simulink model "UART"  (R2025a)
settings: Solver=FixedStepAuto  StartTime=0.0  StopTime=10  FixedStep=1e-6  RelTol=1e-3
undefined symbols (not defined in the file): Bit_1, Bit_2, Bit_3, Bit_4, Bit_5, Bit_6, Bit_7, Bit_8
libraries: simulink_extras x158, fl_lib x17, nesl_utility x8, simulink x7
(part 2 of 6)

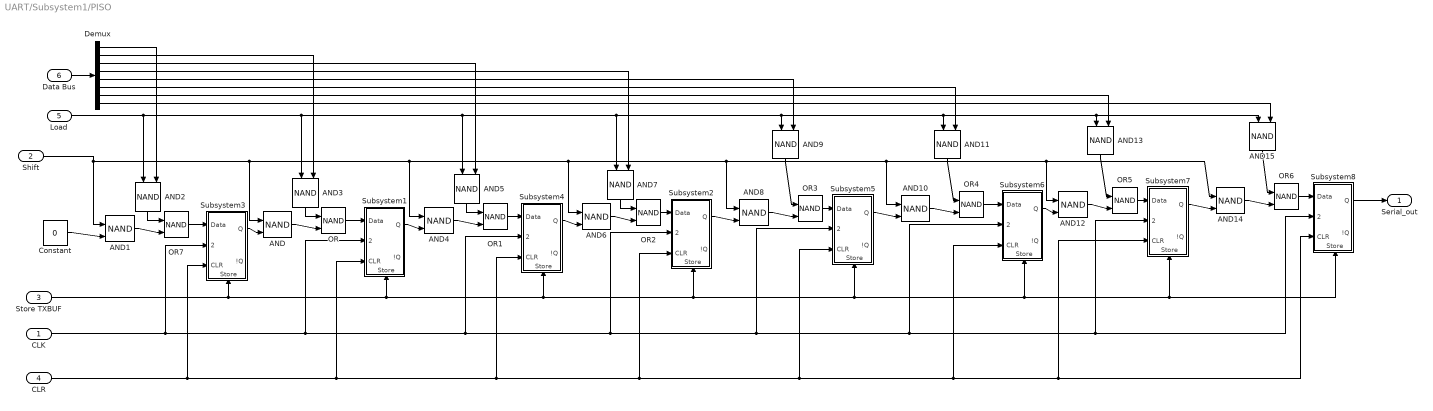
== system UART/Subsystem1/PISO ==
  "CLK " : Inport
  Shift : Inport  Port=2
  Store TXBUF : Inport  Port=3
  "CLR " : Inport  Port=4
  Load : Inport  Port=5
  Data Bus : Inport  Port=6
  AND{,1..15} (16 alike) : Logic  Operator=NAND  IconShape=distinctive  AllPortsSameDT=off  OutDataTypeStr=boolean
  Constant : Constant  Value=0
  Demux : Demux  Outputs=8
  OR{,1..7} (8 alike) : Logic  Operator=NAND  IconShape=distinctive  AllPortsSameDT=off  OutDataTypeStr=boolean
  Subsystem1 : Subsystem
      settings: PortSchema="{\"entries\":[{\"content\":{\"sides\":[{\"content\":{\"connectorIds\":[\"In1\",\"In2\",\"In3\"]},\"type\":\"ConnectorPlacement.EquallySpacedRectSide\",\"uuid\":\"7f3c85a8-435a-48c3-b59c-f5d5714c847e\"},{\"content\":{\"connectorIds\":[\"Out1\",\"Out2\"],\"side\":\"RIGHT\"},\"type\":\"ConnectorPlacement.EquallySpacedRectSide\",\"uuid\":\"17207f13-8340-45d6-91b4-1610668ce323\"},{\"content\":{\"side\":\"TOP\"},\"type\":\"ConnectorPlacement.EquallySpacedRectSide\",\"uuid\":\"04d61695-a4c9-4852-a4b1-2cdbdbfa921f\"},{\"content\":{\"connectorIds\":[\"In4\"],\"side\":\"BOTTOM\"},\"type\":\"ConnectorPlacement.EquallySpacedRectSide\",\"uuid\":\"a1770489-59eb-478b-9b54-00148a18765c\"}]},\"type\":\"ConnectorPlacement.EquallySpacedConnector\",\"uuid\":\"06dc9f9c-9f45-42f3-b967-f8303bc685fc\"}],\"packageUris\":[\"http://schema.mathworks.com/mf0/Connector/R2020b\"],\"version\":\"1.0\"}"
  Subsystem2 : Subsystem
      settings: PortSchema="{\"entries\":[{\"content\":{\"sides\":[{\"content\":{\"connectorIds\":[\"In1\",\"In2\",\"In3\"]},\"type\":\"ConnectorPlacement.EquallySpacedRectSide\",\"uuid\":\"7f3c85a8-435a-48c3-b59c-f5d5714c847e\"},{\"content\":{\"connectorIds\":[\"Out1\",\"Out2\"],\"side\":\"RIGHT\"},\"type\":\"ConnectorPlacement.EquallySpacedRectSide\",\"uuid\":\"17207f13-8340-45d6-91b4-1610668ce323\"},{\"content\":{\"side\":\"TOP\"},\"type\":\"ConnectorPlacement.EquallySpacedRectSide\",\"uuid\":\"04d61695-a4c9-4852-a4b1-2cdbdbfa921f\"},{\"content\":{\"connectorIds\":[\"In4\"],\"side\":\"BOTTOM\"},\"type\":\"ConnectorPlacement.EquallySpacedRectSide\",\"uuid\":\"a1770489-59eb-478b-9b54-00148a18765c\"}]},\"type\":\"ConnectorPlacement.EquallySpacedConnector\",\"uuid\":\"06dc9f9c-9f45-42f3-b967-f8303bc685fc\"}],\"packageUris\":[\"http://schema.mathworks.com/mf0/Connector/R2020b\"],\"version\":\"1.0\"}"
  Subsystem3 : Subsystem
      settings: PortSchema="{\"entries\":[{\"content\":{\"sides\":[{\"content\":{\"connectorIds\":[\"In1\",\"In2\",\"In3\"]},\"type\":\"ConnectorPlacement.EquallySpacedRectSide\",\"uuid\":\"7f3c85a8-435a-48c3-b59c-f5d5714c847e\"},{\"content\":{\"connectorIds\":[\"Out1\",\"Out2\"],\"side\":\"RIGHT\"},\"type\":\"ConnectorPlacement.EquallySpacedRectSide\",\"uuid\":\"17207f13-8340-45d6-91b4-1610668ce323\"},{\"content\":{\"side\":\"TOP\"},\"type\":\"ConnectorPlacement.EquallySpacedRectSide\",\"uuid\":\"04d61695-a4c9-4852-a4b1-2cdbdbfa921f\"},{\"content\":{\"connectorIds\":[\"In4\"],\"side\":\"BOTTOM\"},\"type\":\"ConnectorPlacement.EquallySpacedRectSide\",\"uuid\":\"a1770489-59eb-478b-9b54-00148a18765c\"}]},\"type\":\"ConnectorPlacement.EquallySpacedConnector\",\"uuid\":\"06dc9f9c-9f45-42f3-b967-f8303bc685fc\"}],\"packageUris\":[\"http://schema.mathworks.com/mf0/Connector/R2020b\"],\"version\":\"1.0\"}"
  Subsystem4 : Subsystem
      settings: PortSchema="{\"entries\":[{\"content\":{\"sides\":[{\"content\":{\"connectorIds\":[\"In1\",\"In2\",\"In3\"]},\"type\":\"ConnectorPlacement.EquallySpacedRectSide\",\"uuid\":\"7f3c85a8-435a-48c3-b59c-f5d5714c847e\"},{\"content\":{\"connectorIds\":[\"Out1\",\"Out2\"],\"side\":\"RIGHT\"},\"type\":\"ConnectorPlacement.EquallySpacedRectSide\",\"uuid\":\"17207f13-8340-45d6-91b4-1610668ce323\"},{\"content\":{\"side\":\"TOP\"},\"type\":\"ConnectorPlacement.EquallySpacedRectSide\",\"uuid\":\"04d61695-a4c9-4852-a4b1-2cdbdbfa921f\"},{\"content\":{\"connectorIds\":[\"In4\"],\"side\":\"BOTTOM\"},\"type\":\"ConnectorPlacement.EquallySpacedRectSide\",\"uuid\":\"a1770489-59eb-478b-9b54-00148a18765c\"}]},\"type\":\"ConnectorPlacement.EquallySpacedConnector\",\"uuid\":\"06dc9f9c-9f45-42f3-b967-f8303bc685fc\"}],\"packageUris\":[\"http://schema.mathworks.com/mf0/Connector/R2020b\"],\"version\":\"1.0\"}"
  Subsystem5 : Subsystem
      settings: PortSchema="{\"entries\":[{\"content\":{\"sides\":[{\"content\":{\"connectorIds\":[\"In1\",\"In2\",\"In3\"]},\"type\":\"ConnectorPlacement.EquallySpacedRectSide\",\"uuid\":\"7f3c85a8-435a-48c3-b59c-f5d5714c847e\"},{\"content\":{\"connectorIds\":[\"Out1\",\"Out2\"],\"side\":\"RIGHT\"},\"type\":\"ConnectorPlacement.EquallySpacedRectSide\",\"uuid\":\"17207f13-8340-45d6-91b4-1610668ce323\"},{\"content\":{\"side\":\"TOP\"},\"type\":\"ConnectorPlacement.EquallySpacedRectSide\",\"uuid\":\"04d61695-a4c9-4852-a4b1-2cdbdbfa921f\"},{\"content\":{\"connectorIds\":[\"In4\"],\"side\":\"BOTTOM\"},\"type\":\"ConnectorPlacement.EquallySpacedRectSide\",\"uuid\":\"a1770489-59eb-478b-9b54-00148a18765c\"}]},\"type\":\"ConnectorPlacement.EquallySpacedConnector\",\"uuid\":\"06dc9f9c-9f45-42f3-b967-f8303bc685fc\"}],\"packageUris\":[\"http://schema.mathworks.com/mf0/Connector/R2020b\"],\"version\":\"1.0\"}"
  Subsystem6 : Subsystem
      settings: PortSchema="{\"entries\":[{\"content\":{\"sides\":[{\"content\":{\"connectorIds\":[\"In1\",\"In2\",\"In3\"]},\"type\":\"ConnectorPlacement.EquallySpacedRectSide\",\"uuid\":\"7f3c85a8-435a-48c3-b59c-f5d5714c847e\"},{\"content\":{\"connectorIds\":[\"Out1\",\"Out2\"],\"side\":\"RIGHT\"},\"type\":\"ConnectorPlacement.EquallySpacedRectSide\",\"uuid\":\"17207f13-8340-45d6-91b4-1610668ce323\"},{\"content\":{\"side\":\"TOP\"},\"type\":\"ConnectorPlacement.EquallySpacedRectSide\",\"uuid\":\"04d61695-a4c9-4852-a4b1-2cdbdbfa921f\"},{\"content\":{\"connectorIds\":[\"In4\"],\"side\":\"BOTTOM\"},\"type\":\"ConnectorPlacement.EquallySpacedRectSide\",\"uuid\":\"a1770489-59eb-478b-9b54-00148a18765c\"}]},\"type\":\"ConnectorPlacement.EquallySpacedConnector\",\"uuid\":\"06dc9f9c-9f45-42f3-b967-f8303bc685fc\"}],\"packageUris\":[\"http://schema.mathworks.com/mf0/Connector/R2020b\"],\"version\":\"1.0\"}"
  Subsystem7 : Subsystem
      settings: PortSchema="{\"entries\":[{\"content\":{\"sides\":[{\"content\":{\"connectorIds\":[\"In1\",\"In2\",\"In3\"]},\"type\":\"ConnectorPlacement.EquallySpacedRectSide\",\"uuid\":\"7f3c85a8-435a-48c3-b59c-f5d5714c847e\"},{\"content\":{\"connectorIds\":[\"Out1\",\"Out2\"],\"side\":\"RIGHT\"},\"type\":\"ConnectorPlacement.EquallySpacedRectSide\",\"uuid\":\"17207f13-8340-45d6-91b4-1610668ce323\"},{\"content\":{\"side\":\"TOP\"},\"type\":\"ConnectorPlacement.EquallySpacedRectSide\",\"uuid\":\"04d61695-a4c9-4852-a4b1-2cdbdbfa921f\"},{\"content\":{\"connectorIds\":[\"In4\"],\"side\":\"BOTTOM\"},\"type\":\"ConnectorPlacement.EquallySpacedRectSide\",\"uuid\":\"a1770489-59eb-478b-9b54-00148a18765c\"}]},\"type\":\"ConnectorPlacement.EquallySpacedConnector\",\"uuid\":\"06dc9f9c-9f45-42f3-b967-f8303bc685fc\"}],\"packageUris\":[\"http://schema.mathworks.com/mf0/Connector/R2020b\"],\"version\":\"1.0\"}"
  Subsystem8 : Subsystem
      settings: PortSchema="{\"entries\":[{\"content\":{\"sides\":[{\"content\":{\"connectorIds\":[\"In1\",\"In2\",\"In3\"]},\"type\":\"ConnectorPlacement.EquallySpacedRectSide\",\"uuid\":\"7f3c85a8-435a-48c3-b59c-f5d5714c847e\"},{\"content\":{\"connectorIds\":[\"Out1\",\"Out2\"],\"side\":\"RIGHT\"},\"type\":\"ConnectorPlacement.EquallySpacedRectSide\",\"uuid\":\"17207f13-8340-45d6-91b4-1610668ce323\"},{\"content\":{\"side\":\"TOP\"},\"type\":\"ConnectorPlacement.EquallySpacedRectSide\",\"uuid\":\"04d61695-a4c9-4852-a4b1-2cdbdbfa921f\"},{\"content\":{\"connectorIds\":[\"In4\"],\"side\":\"BOTTOM\"},\"type\":\"ConnectorPlacement.EquallySpacedRectSide\",\"uuid\":\"a1770489-59eb-478b-9b54-00148a18765c\"}]},\"type\":\"ConnectorPlacement.EquallySpacedConnector\",\"uuid\":\"06dc9f9c-9f45-42f3-b967-f8303bc685fc\"}],\"packageUris\":[\"http://schema.mathworks.com/mf0/Connector/R2020b\"],\"version\":\"1.0\"}"
  Serial_out : Outport
  wires:
  AND12/1 -> OR5/2
  AND14/1 -> OR6/2
  AND13/1 -> OR5/1
  OR6/1 -> Subsystem8/1(Data)
  AND6/1 -> OR2/2
  AND7/1 -> OR2/1
  Subsystem4/1(Q) -> AND6/2
  OR2/1 -> Subsystem2/1(Data)
  Subsystem2/1(Q) -> AND8/2
  AND15/1 -> OR6/1
  AND8/1 -> OR3/2
  AND3/1 -> OR/1
  OR5/1 -> Subsystem7/1(Data)
  Subsystem7/1(Q) -> AND14/2
  AND11/1 -> OR4/1
  AND9/1 -> OR3/1
  Subsystem6/1(Q) -> AND12/2
  OR3/1 -> Subsystem5/1(Data)
  OR4/1 -> Subsystem6/1(Data)
  OR1/1 -> Subsystem4/1(Data)
  AND5/1 -> OR1/1
  AND/1 -> OR/2
  AND4/1 -> OR1/2
  Subsystem1/1(Q) -> AND4/2
  Subsystem3/1(Q) -> AND/2
  OR/1 -> Subsystem1/1(Data)
  OR7/1 -> Subsystem3/1(Data)
  Subsystem5/1(Q) -> AND10/2
  AND10/1 -> OR4/2
  Data Bus/1 -> Demux/1
  AND2/1 -> OR7/1
  AND1/1 -> OR7/2
  Shift/1 -> AND1/1, AND6/1, AND10/1, AND12/1, AND14/1, AND8/1, AND4/1, AND/1
  Subsystem8/1(Q) -> Serial_out/1
  Store TXBUF/1 -> Subsystem3/4(Store), Subsystem1/4(Store), Subsystem4/4(Store), Subsystem2/4(Store), Subsystem5/4(Store), Subsystem6/4(Store), Subsystem8/4(Store), Subsystem7/4(Store)
  "CLK "/1 -> Subsystem3/2(Clock), Subsystem1/2(Clock), Subsystem4/2(Clock), Subsystem2/2(Clock), Subsystem5/2(Clock), Subsystem6/2(Clock), Subsystem8/2(Clock), Subsystem7/2(Clock)
  "CLR "/1 -> Subsystem3/3(CLR), Subsystem1/3(CLR), Subsystem4/3(CLR), Subsystem2/3(CLR), Subsystem5/3(CLR), Subsystem6/3(CLR), Subsystem8/3(CLR), Subsystem7/3(CLR)
  Constant/1 -> AND1/2
  Load/1 -> AND2/1, AND3/1, AND5/1, AND7/1, AND9/1, AND11/1, AND13/1, AND15/1
  Demux/1 -> AND2/2
  Demux/2 -> AND3/2
  Demux/3 -> AND5/2
  Demux/4 -> AND7/2
  Demux/5 -> AND9/2
  Demux/6 -> AND11/2
  Demux/7 -> AND13/2
  Demux/8 -> AND15/2

== system UART/Subsystem1/RX Counter ==
  BC_Reset : Inport
  INC : Inport  Port=2
  Constant : Constant
  D Flip-Flop{5..7,11} (4 alike) : simulink_extras/Flip Flops/D Flip-Flop
  Delay One Step : Delay  DelayLength=1
  Demux : Demux
  Half Adder : Subsystem
      settings: PortSchema="{\"entries\":[{\"content\":{\"sides\":[{\"content\":{\"connectorIds\":[\"In1\"]},\"type\":\"ConnectorPlacement.EquallySpacedRectSide\",\"uuid\":\"d3a7e232-15f2-47a9-a065-9480c81dc57e\"},{\"content\":{\"connectorIds\":[\"Out1\"],\"side\":\"RIGHT\"},\"type\":\"ConnectorPlacement.EquallySpacedRectSide\",\"uuid\":\"e118f150-fee7-4aeb-941e-53c3f02c6791\"},{\"content\":{\"connectorIds\":[\"Out2\"],\"side\":\"TOP\"},\"type\":\"ConnectorPlacement.EquallySpacedRectSide\",\"uuid\":\"6d9038ab-faad-455b-a9c5-8fe0bbf34e51\"},{\"content\":{\"connectorIds\":[\"In2\"],\"side\":\"BOTTOM\"},\"type\":\"ConnectorPlacement.EquallySpacedRectSide\",\"uuid\":\"d09c8d4f-08f3-4c52-88a6-8c6db517fc7a\"}]},\"type\":\"ConnectorPlacement.EquallySpacedConnector\",\"uuid\":\"5bc947ce-f1cd-4957-9186-40c14c78de7d\"}],\"packageUris\":[\"http://schema.mathworks.com/mf0/Connector/R2020b\"],\"version\":\"1.0\"}"
  Half Adder1 : Subsystem
      settings: PortSchema="{\"entries\":[{\"content\":{\"sides\":[{\"content\":{\"connectorIds\":[\"In1\"]},\"type\":\"ConnectorPlacement.EquallySpacedRectSide\",\"uuid\":\"d3a7e232-15f2-47a9-a065-9480c81dc57e\"},{\"content\":{\"connectorIds\":[\"Out1\"],\"side\":\"RIGHT\"},\"type\":\"ConnectorPlacement.EquallySpacedRectSide\",\"uuid\":\"e118f150-fee7-4aeb-941e-53c3f02c6791\"},{\"content\":{\"connectorIds\":[\"Out2\"],\"side\":\"TOP\"},\"type\":\"ConnectorPlacement.EquallySpacedRectSide\",\"uuid\":\"6d9038ab-faad-455b-a9c5-8fe0bbf34e51\"},{\"content\":{\"connectorIds\":[\"In2\"],\"side\":\"BOTTOM\"},\"type\":\"ConnectorPlacement.EquallySpacedRectSide\",\"uuid\":\"d09c8d4f-08f3-4c52-88a6-8c6db517fc7a\"}]},\"type\":\"ConnectorPlacement.EquallySpacedConnector\",\"uuid\":\"5bc947ce-f1cd-4957-9186-40c14c78de7d\"}],\"packageUris\":[\"http://schema.mathworks.com/mf0/Connector/R2020b\"],\"version\":\"1.0\"}"
  Half Adder2 : Subsystem
      settings: PortSchema="{\"entries\":[{\"content\":{\"sides\":[{\"content\":{\"connectorIds\":[\"In1\"]},\"type\":\"ConnectorPlacement.EquallySpacedRectSide\",\"uuid\":\"d3a7e232-15f2-47a9-a065-9480c81dc57e\"},{\"content\":{\"connectorIds\":[\"Out1\"],\"side\":\"RIGHT\"},\"type\":\"ConnectorPlacement.EquallySpacedRectSide\",\"uuid\":\"e118f150-fee7-4aeb-941e-53c3f02c6791\"},{\"content\":{\"connectorIds\":[\"Out2\"],\"side\":\"TOP\"},\"type\":\"ConnectorPlacement.EquallySpacedRectSide\",\"uuid\":\"6d9038ab-faad-455b-a9c5-8fe0bbf34e51\"},{\"content\":{\"connectorIds\":[\"In2\"],\"side\":\"BOTTOM\"},\"type\":\"ConnectorPlacement.EquallySpacedRectSide\",\"uuid\":\"d09c8d4f-08f3-4c52-88a6-8c6db517fc7a\"}]},\"type\":\"ConnectorPlacement.EquallySpacedConnector\",\"uuid\":\"5bc947ce-f1cd-4957-9186-40c14c78de7d\"}],\"packageUris\":[\"http://schema.mathworks.com/mf0/Connector/R2020b\"],\"version\":\"1.0\"}"
  Half Adder7 : Subsystem
      settings: PortSchema="{\"entries\":[{\"content\":{\"sides\":[{\"content\":{\"connectorIds\":[\"In1\"]},\"type\":\"ConnectorPlacement.EquallySpacedRectSide\",\"uuid\":\"d3a7e232-15f2-47a9-a065-9480c81dc57e\"},{\"content\":{\"connectorIds\":[\"Out1\"],\"side\":\"RIGHT\"},\"type\":\"ConnectorPlacement.EquallySpacedRectSide\",\"uuid\":\"e118f150-fee7-4aeb-941e-53c3f02c6791\"},{\"content\":{\"connectorIds\":[\"Out2\"],\"side\":\"TOP\"},\"type\":\"ConnectorPlacement.EquallySpacedRectSide\",\"uuid\":\"6d9038ab-faad-455b-a9c5-8fe0bbf34e51\"},{\"content\":{\"connectorIds\":[\"In2\"],\"side\":\"BOTTOM\"},\"type\":\"ConnectorPlacement.EquallySpacedRectSide\",\"uuid\":\"d09c8d4f-08f3-4c52-88a6-8c6db517fc7a\"}]},\"type\":\"ConnectorPlacement.EquallySpacedConnector\",\"uuid\":\"5bc947ce-f1cd-4957-9186-40c14c78de7d\"}],\"packageUris\":[\"http://schema.mathworks.com/mf0/Connector/R2020b\"],\"version\":\"1.0\"}"
  Mux1 : Mux
  NOT : Logic  Operator=NOT  IconShape=distinctive  AllPortsSameDT=off  OutDataTypeStr=boolean
  C4 : Outport
  !C3 : Outport  Port=2
  !C2 : Outport  Port=3
  C1 : Outport  Port=4
  C2 : Outport  Port=5
  !C1 : Outport  Port=6
  wires:
  Mux1/1 -> Delay One Step/1
  BC_Reset/1 -> NOT/1
  Delay One Step/1 -> Demux/1
  Demux/4 -> D Flip-Flop7/1
  Demux/3 -> D Flip-Flop5/1
  Demux/2 -> D Flip-Flop6/1
  Demux/1 -> D Flip-Flop11/1
  INC/1 -> D Flip-Flop11/2, D Flip-Flop6/2, D Flip-Flop5/2, D Flip-Flop7/2
  Constant/1 -> Half Adder7/2("B ")
  Half Adder/2(Carry) -> Half Adder1/2("B ")
  Half Adder1/1(Sum) -> Mux1/2
  Half Adder/1(Sum) -> Mux1/3
  Half Adder2/1(Sum) -> Mux1/1
  Half Adder1/2(Carry) -> Half Adder2/2("B ")
  Half Adder7/1(Sum) -> Mux1/4
  Half Adder7/2(Carry) -> Half Adder/2("B ")
  D Flip-Flop11/1 -> C4/1, Half Adder2/1(A)  "D1"
  D Flip-Flop6/1 -> Half Adder1/1(A)  "D3"
  D Flip-Flop5/1 -> C2/1, Half Adder/1(A)  "D4"
  D Flip-Flop7/1 -> C1/1, Half Adder7/1(A)  "D2"
  NOT/1 -> D Flip-Flop11/3, D Flip-Flop6/3, D Flip-Flop5/3, D Flip-Flop7/3
  D Flip-Flop5/2 -> !C2/1
  D Flip-Flop6/2 -> !C3/1
  D Flip-Flop7/2 -> !C1/1

== system UART/Subsystem1/SISO RxBuf ==
  Rx : Inport
  CLK : Inport  Port=2
  Constant : Constant
  D Flip-Flop{,1..7} (8 alike) : simulink_extras/Flip Flops/D Flip-Flop
  Mux : Mux  Inputs=8
  RxBuf : Outport
  wires:
  D Flip-Flop4/1 -> D Flip-Flop5/1, Mux/5
  Constant/1 -> D Flip-Flop6/3, D Flip-Flop7/3, D Flip-Flop5/3, D Flip-Flop4/3, D Flip-Flop3/3, D Flip-Flop2/3, D Flip-Flop1/3, D Flip-Flop/3
  Mux/1 -> RxBuf/1
  CLK/1 -> D Flip-Flop1/2, D Flip-Flop2/2, D Flip-Flop3/2, D Flip-Flop4/2, D Flip-Flop5/2, D Flip-Flop6/2, D Flip-Flop7/2, D Flip-Flop/2
  D Flip-Flop6/1 -> D Flip-Flop7/1, Mux/7
  D Flip-Flop1/1 -> D Flip-Flop2/1, Mux/2
  D Flip-Flop2/1 -> D Flip-Flop3/1, Mux/3
  D Flip-Flop3/2 -> ?
  D Flip-Flop3/1 -> D Flip-Flop4/1, Mux/4
  D Flip-Flop7/1 -> Mux/8
  D Flip-Flop/1 -> D Flip-Flop1/1, Mux/1
  D Flip-Flop5/1 -> D Flip-Flop6/1, Mux/6
  D Flip-Flop2/2 -> ?
  Rx/1 -> D Flip-Flop/1

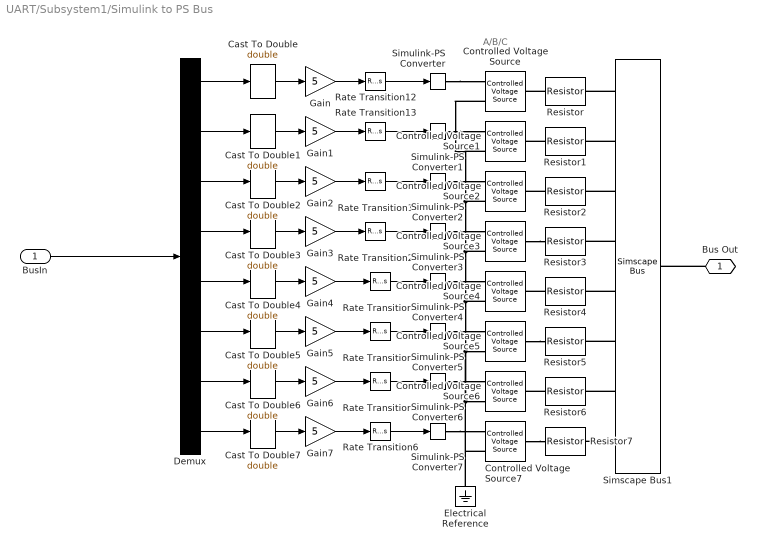
== system UART/Subsystem1/Simulink to PS Bus ==
  note: A/B/C
  BusIn : Inport
  Cast To Double{,1..7} (8 alike) : DataTypeConversion  OutDataTypeStr=double  SaturateOnIntegerOverflow=off  RndMeth=Floor
  Controlled Voltage Source{,1..7} (8 alike) : fl_lib/Electrical/Electrical Sources/Controlled Voltage Source
  Demux : Demux  Outputs=8
  Electrical Reference : fl_lib/Electrical/Electrical Elements/Electrical Reference
  Gain{,1..7} (8 alike) : Gain  Gain=5
  Rate Transition{1..6,12..13} (8 alike) : RateTransition
  Resistor{,1..7} (8 alike) : fl_lib/Electrical/Electrical Elements/Resistor  R=1 Ohm  i_specify=off  i_priority=None  i=0 A  i_nominal_specify=off  i_nominal_value=1  i_nominal_unit=A  v_specify=off  v_priority=None  v=0 V  v_nominal_specify=off  v_nominal_value=1  v_nominal_unit=V
  Simscape Bus1 : SimscapeBus  HierarchyStrings=Bit_8;Bit_7;Bit_6;Bit_5;Bit_4;Bit_3;Bit_2;Bit_1
  Simulink-PS Converter{,1..7} (8 alike) : nesl_utility/Simulink-PS Converter  PhysicalDomain=network_engine_domain  SubClassName=ps_input  LeftPortType=input  RightPortType=output  PseudoPeriodic=off  Frequencies=[]  NoiseDistribution=none  NoiseParameters=[]  Unit=1  AffineConversion=off  FilteringAndDerivatives=provide  SimscapeFilterOrder=1  InputFilterTimeConstant=0.001  UdotUserProvided=0
  Bus Out : PMIOPort  Side=Right
  wires:
  BusIn/1 -> Demux/1
  Demux/5 -> Cast To Double4/1
  Cast To Double5/1 -> Gain5/1
  Cast To Double6/1 -> Gain6/1
  Cast To Double7/1 -> Gain7/1
  Gain/1 -> Rate Transition12/1
  Demux/2 -> Cast To Double1/1
  Demux/4 -> Cast To Double3/1
  Gain5/1 -> Rate Transition5/1
  Gain4/1 -> Rate Transition4/1
  Gain2/1 -> Rate Transition1/1
  Cast To Double2/1 -> Gain2/1
  Cast To Double4/1 -> Gain4/1
  Gain6/1 -> Rate Transition3/1
  Cast To Double3/1 -> Gain3/1
  Cast To Double/1 -> Gain/1
  Cast To Double1/1 -> Gain1/1
  Demux/7 -> Cast To Double6/1
  Demux/1 -> Cast To Double/1
  Gain3/1 -> Rate Transition2/1
  Demux/6 -> Cast To Double5/1
  Gain7/1 -> Rate Transition6/1
  Demux/8 -> Cast To Double7/1
  Demux/3 -> Cast To Double2/1
  Gain1/1 -> Rate Transition13/1
  Rate Transition12/1 -> Simulink-PS Converter/1
  Rate Transition13/1 -> Simulink-PS Converter1/1
  Rate Transition1/1 -> Simulink-PS Converter2/1
  Rate Transition2/1 -> Simulink-PS Converter3/1
  Rate Transition6/1 -> Simulink-PS Converter7/1
  Rate Transition4/1 -> Simulink-PS Converter4/1
  Rate Transition3/1 -> Simulink-PS Converter6/1
  Rate Transition5/1 -> Simulink-PS Converter5/1
  connections:
  Controlled Voltage Source2/RConn2 -- Controlled Voltage Source/RConn2 -- Controlled Voltage Source1/RConn2 -- Controlled Voltage Source5/RConn2 -- Electrical Reference/LConn1 -- Controlled Voltage Source7/RConn2 -- Controlled Voltage Source6/RConn2 -- Controlled Voltage Source4/RConn2 -- Controlled Voltage Source3/RConn2
  Simscape Bus1/LConn7 -- Resistor6/RConn1
  Simscape Bus1/LConn5 -- Resistor4/RConn1
  Simscape Bus1/LConn8 -- Resistor7/RConn1
  Simulink-PS Converter5/RConn1 -- Controlled Voltage Source5/RConn1
  Simulink-PS Converter4/RConn1 -- Controlled Voltage Source4/RConn1
  Simulink-PS Converter6/RConn1 -- Controlled Voltage Source6/RConn1
  Simulink-PS Converter/RConn1 -- Controlled Voltage Source/RConn1
  Simulink-PS Converter1/RConn1 -- Controlled Voltage Source1/RConn1
  Simscape Bus1/LConn4 -- Resistor3/RConn1
  Controlled Voltage Source5/LConn1 -- Resistor5/LConn1
  Simulink-PS Converter7/RConn1 -- Controlled Voltage Source7/RConn1
  Simulink-PS Converter3/RConn1 -- Controlled Voltage Source3/RConn1
  Simscape Bus1/LConn2 -- Resistor1/RConn1
  Simulink-PS Converter2/RConn1 -- Controlled Voltage Source2/RConn1
  Resistor2/LConn1 -- Controlled Voltage Source2/LConn1
  Resistor/LConn1 -- Controlled Voltage Source/LConn1
  Simscape Bus1/LConn1 -- Resistor/RConn1
  Resistor1/LConn1 -- Controlled Voltage Source1/LConn1
  Simscape Bus1/LConn3 -- Resistor2/RConn1
  Controlled Voltage Source3/LConn1 -- Resistor3/LConn1
  Resistor4/LConn1 -- Controlled Voltage Source4/LConn1
  Simscape Bus1/LConn6 -- Resistor5/RConn1
  Resistor6/LConn1 -- Controlled Voltage Source6/LConn1
  Controlled Voltage Source7/LConn1 -- Resistor7/LConn1
  Bus Out/RConn1 -- Simscape Bus1/RConn1

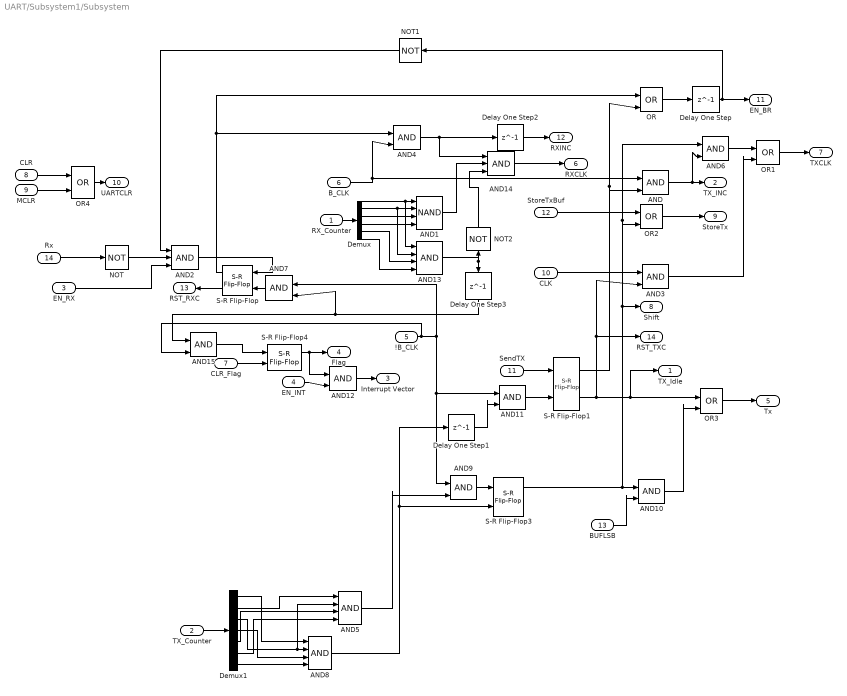
== system UART/Subsystem1/Subsystem ==
  RX_Counter : Inport
  TX_Counter : Inport  Port=2
  EN_RX : Inport  Port=3
  EN_INT : Inport  Port=4
  !B_CLK : Inport  Port=5
  B_CLK : Inport  Port=6
  CLR_Flag : Inport  Port=7
  CLR : Inport  Port=8
  MCLR : Inport  Port=9
  CLK : Inport  Port=10
  SendTX : Inport  Port=11
  StoreTxBuf : Inport  Port=12
  BUFLSB : Inport  Port=13
  Rx : Inport  Port=14
  AND{,3..4,6..7,9..12,15} (10 alike) : Logic  IconShape=distinctive  AllPortsSameDT=off  OutDataTypeStr=boolean
  AND1 : Logic  Operator=NAND  Inputs=4  IconShape=distinctive  AllPortsSameDT=off  OutDataTypeStr=boolean
  AND13 : Logic  Inputs=4  IconShape=distinctive  AllPortsSameDT=off  OutDataTypeStr=boolean
  AND14 : Logic  Inputs=3  IconShape=distinctive  AllPortsSameDT=off  OutDataTypeStr=boolean
  AND2 : Logic  Inputs=3  IconShape=distinctive  AllPortsSameDT=off  OutDataTypeStr=boolean
  AND5 : Logic  Inputs=4  IconShape=distinctive  AllPortsSameDT=off  OutDataTypeStr=boolean
  AND8 : Logic  Inputs=4  IconShape=distinctive  AllPortsSameDT=off  OutDataTypeStr=boolean
  Delay One Step : Delay  DelayLength=1
  Delay One Step1 : Delay  DelayLength=1  SampleTime=1e-5
  Delay One Step2 : Delay  DelayLength=1
  Delay One Step3 : Delay  DelayLength=1
  Demux : Demux  Outputs=6
  Demux1 : Demux  Outputs=7
  NOT : Logic  Operator=NOT  IconShape=distinctive  AllPortsSameDT=off  OutDataTypeStr=boolean
  NOT1 : Logic  Operator=NOT  IconShape=distinctive  AllPortsSameDT=off  OutDataTypeStr=boolean
  NOT2 : Logic  Operator=NOT  IconShape=distinctive  AllPortsSameDT=off  OutDataTypeStr=boolean
  OR{,1..4} (5 alike) : Logic  Operator=OR  IconShape=distinctive  AllPortsSameDT=off  OutDataTypeStr=boolean
  S-R Flip-Flop{,1,3..4} (4 alike) : simulink_extras/Flip Flops/S-R Flip-Flop  initial_condition=0
  TX_Idle : Outport
  TX_INC : Outport  Port=2
  Interrupt Vector : Outport  Port=3
  Flag : Outport  Port=4
  Tx : Outport  Port=5
  RXCLK : Outport  Port=6
  TXCLK : Outport  Port=7
  Shift : Outport  Port=8
  StoreTx : Outport  Port=9
  UARTCLR : Outport  Port=10
  EN_BR : Outport  Port=11
  RXINC : Outport  Port=12
  RST_RXC : Outport  Port=13
  RST_TXC : Outport  Port=14
  wires:
  Rx/1 -> NOT/1
  OR4/1 -> UARTCLR/1
  !B_CLK/1 -> AND15/2, AND9/1, AND11/1, AND7/1
  NOT/1 -> AND2/2
  EN_RX/1 -> AND2/3
  AND2/1 -> S-R Flip-Flop/1
  EN_INT/1 -> AND12/2
  S-R Flip-Flop4/1 -> AND12/1, Flag/1
  AND12/1 -> Interrupt Vector/1
  CLR_Flag/1 -> S-R Flip-Flop4/2
  S-R Flip-Flop/2 -> RST_RXC/1
  Demux/1 -> AND13/1, AND1/1
  Demux/2 -> AND13/2, AND1/2
  Demux/3 -> AND1/3
  Demux/4 -> AND1/4
  B_CLK/1 -> AND4/2, AND/1
  OR2/1 -> StoreTx/1
  AND3/1 -> OR1/2
  S-R Flip-Flop1/2 -> AND3/2, RST_TXC/1, TX_Idle/1, OR3/1
  CLK/1 -> AND3/1
  AND4/1 -> Delay One Step2/1, AND14/1
  S-R Flip-Flop1/1 -> OR/2, AND/2
  AND8/1 -> Delay One Step1/1, S-R Flip-Flop3/2
  AND5/1 -> AND9/2
  AND1/1 -> AND14/2
  OR1/1 -> TXCLK/1
  Delay One Step1/1 -> AND11/2
  AND9/1 -> S-R Flip-Flop3/1
  SendTX/1 -> S-R Flip-Flop1/1
  AND11/1 -> S-R Flip-Flop1/2
  S-R Flip-Flop3/1 -> AND10/1, AND6/1, OR2/2, Shift/1
  StoreTxBuf/1 -> OR2/1
  BUFLSB/1 -> AND10/2
  AND/1 -> AND6/2, TX_INC/1
  AND10/1 -> OR3/2
  AND6/1 -> OR1/1
  OR3/1 -> Tx/1
  RX_Counter/1 -> Demux/1
  TX_Counter/1 -> Demux1/1
  CLR/1 -> OR4/1
  MCLR/1 -> OR4/2
  OR/1 -> Delay One Step/1
  Demux1/7 -> AND8/4
  Demux1/4 -> AND8/3
  Demux1/3 -> AND5/2, AND8/2
  Demux1/1 -> AND8/1
  Demux1/6 -> AND5/4
  Demux1/5 -> AND5/3
  Demux1/2 -> AND5/1
  Delay One Step/1 -> NOT1/1, EN_BR/1
  Delay One Step3/1 -> AND15/1, AND7/2
  AND7/1 -> S-R Flip-Flop/2
  NOT1/1 -> AND2/1
  S-R Flip-Flop/1 -> OR/1, AND4/1
  Demux/5 -> AND13/3
  Demux/6 -> AND13/4
  AND13/1 -> NOT2/1, Delay One Step3/1
  Delay One Step2/1 -> RXINC/1
  AND14/1 -> RXCLK/1
  NOT2/1 -> AND14/3
  AND15/1 -> S-R Flip-Flop4/1

== system UART/Subsystem1/TX Counter ==
  BC_Reset : Inport
  INC : Inport  Port=2
  Constant : Constant
  D Flip-Flop{5..7,11} (4 alike) : simulink_extras/Flip Flops/D Flip-Flop
  Delay One Step : Delay  DelayLength=1
  Demux : Demux
  Half Adder : Subsystem
      settings: PortSchema="{\"entries\":[{\"content\":{\"sides\":[{\"content\":{\"connectorIds\":[\"In1\"]},\"type\":\"ConnectorPlacement.EquallySpacedRectSide\",\"uuid\":\"d3a7e232-15f2-47a9-a065-9480c81dc57e\"},{\"content\":{\"connectorIds\":[\"Out1\"],\"side\":\"RIGHT\"},\"type\":\"ConnectorPlacement.EquallySpacedRectSide\",\"uuid\":\"e118f150-fee7-4aeb-941e-53c3f02c6791\"},{\"content\":{\"connectorIds\":[\"Out2\"],\"side\":\"TOP\"},\"type\":\"ConnectorPlacement.EquallySpacedRectSide\",\"uuid\":\"6d9038ab-faad-455b-a9c5-8fe0bbf34e51\"},{\"content\":{\"connectorIds\":[\"In2\"],\"side\":\"BOTTOM\"},\"type\":\"ConnectorPlacement.EquallySpacedRectSide\",\"uuid\":\"d09c8d4f-08f3-4c52-88a6-8c6db517fc7a\"}]},\"type\":\"ConnectorPlacement.EquallySpacedConnector\",\"uuid\":\"5bc947ce-f1cd-4957-9186-40c14c78de7d\"}],\"packageUris\":[\"http://schema.mathworks.com/mf0/Connector/R2020b\"],\"version\":\"1.0\"}"
  Half Adder1 : Subsystem
      settings: PortSchema="{\"entries\":[{\"content\":{\"sides\":[{\"content\":{\"connectorIds\":[\"In1\"]},\"type\":\"ConnectorPlacement.EquallySpacedRectSide\",\"uuid\":\"d3a7e232-15f2-47a9-a065-9480c81dc57e\"},{\"content\":{\"connectorIds\":[\"Out1\"],\"side\":\"RIGHT\"},\"type\":\"ConnectorPlacement.EquallySpacedRectSide\",\"uuid\":\"e118f150-fee7-4aeb-941e-53c3f02c6791\"},{\"content\":{\"connectorIds\":[\"Out2\"],\"side\":\"TOP\"},\"type\":\"ConnectorPlacement.EquallySpacedRectSide\",\"uuid\":\"6d9038ab-faad-455b-a9c5-8fe0bbf34e51\"},{\"content\":{\"connectorIds\":[\"In2\"],\"side\":\"BOTTOM\"},\"type\":\"ConnectorPlacement.EquallySpacedRectSide\",\"uuid\":\"d09c8d4f-08f3-4c52-88a6-8c6db517fc7a\"}]},\"type\":\"ConnectorPlacement.EquallySpacedConnector\",\"uuid\":\"5bc947ce-f1cd-4957-9186-40c14c78de7d\"}],\"packageUris\":[\"http://schema.mathworks.com/mf0/Connector/R2020b\"],\"version\":\"1.0\"}"
  Half Adder2 : Subsystem
      settings: PortSchema="{\"entries\":[{\"content\":{\"sides\":[{\"content\":{\"connectorIds\":[\"In1\"]},\"type\":\"ConnectorPlacement.EquallySpacedRectSide\",\"uuid\":\"d3a7e232-15f2-47a9-a065-9480c81dc57e\"},{\"content\":{\"connectorIds\":[\"Out1\"],\"side\":\"RIGHT\"},\"type\":\"ConnectorPlacement.EquallySpacedRectSide\",\"uuid\":\"e118f150-fee7-4aeb-941e-53c3f02c6791\"},{\"content\":{\"connectorIds\":[\"Out2\"],\"side\":\"TOP\"},\"type\":\"ConnectorPlacement.EquallySpacedRectSide\",\"uuid\":\"6d9038ab-faad-455b-a9c5-8fe0bbf34e51\"},{\"content\":{\"connectorIds\":[\"In2\"],\"side\":\"BOTTOM\"},\"type\":\"ConnectorPlacement.EquallySpacedRectSide\",\"uuid\":\"d09c8d4f-08f3-4c52-88a6-8c6db517fc7a\"}]},\"type\":\"ConnectorPlacement.EquallySpacedConnector\",\"uuid\":\"5bc947ce-f1cd-4957-9186-40c14c78de7d\"}],\"packageUris\":[\"http://schema.mathworks.com/mf0/Connector/R2020b\"],\"version\":\"1.0\"}"
  Half Adder7 : Subsystem
      settings: PortSchema="{\"entries\":[{\"content\":{\"sides\":[{\"content\":{\"connectorIds\":[\"In1\"]},\"type\":\"ConnectorPlacement.EquallySpacedRectSide\",\"uuid\":\"d3a7e232-15f2-47a9-a065-9480c81dc57e\"},{\"content\":{\"connectorIds\":[\"Out1\"],\"side\":\"RIGHT\"},\"type\":\"ConnectorPlacement.EquallySpacedRectSide\",\"uuid\":\"e118f150-fee7-4aeb-941e-53c3f02c6791\"},{\"content\":{\"connectorIds\":[\"Out2\"],\"side\":\"TOP\"},\"type\":\"ConnectorPlacement.EquallySpacedRectSide\",\"uuid\":\"6d9038ab-faad-455b-a9c5-8fe0bbf34e51\"},{\"content\":{\"connectorIds\":[\"In2\"],\"side\":\"BOTTOM\"},\"type\":\"ConnectorPlacement.EquallySpacedRectSide\",\"uuid\":\"d09c8d4f-08f3-4c52-88a6-8c6db517fc7a\"}]},\"type\":\"ConnectorPlacement.EquallySpacedConnector\",\"uuid\":\"5bc947ce-f1cd-4957-9186-40c14c78de7d\"}],\"packageUris\":[\"http://schema.mathworks.com/mf0/Connector/R2020b\"],\"version\":\"1.0\"}"
  Mux1 : Mux
  NOT : Logic  Operator=NOT  IconShape=distinctive  AllPortsSameDT=off  OutDataTypeStr=boolean
  C4 : Outport
  !C4 : Outport  Port=2
  !C3 : Outport  Port=3
  C2 : Outport  Port=4
  !C2 : Outport  Port=5
  C1 : Outport  Port=6
  !C1 : Outport  Port=7
  wires:
  Mux1/1 -> Delay One Step/1
  BC_Reset/1 -> NOT/1
  Delay One Step/1 -> Demux/1
  Demux/4 -> D Flip-Flop7/1
  Demux/3 -> D Flip-Flop5/1
  Demux/2 -> D Flip-Flop6/1
  Demux/1 -> D Flip-Flop11/1
  INC/1 -> D Flip-Flop11/2, D Flip-Flop6/2, D Flip-Flop5/2, D Flip-Flop7/2
  Constant/1 -> Half Adder7/2("B ")
  Half Adder/2(Carry) -> Half Adder1/2("B ")
  Half Adder1/1(Sum) -> Mux1/2
  Half Adder/1(Sum) -> Mux1/3
  Half Adder2/1(Sum) -> Mux1/1
  Half Adder1/2(Carry) -> Half Adder2/2("B ")
  Half Adder7/1(Sum) -> Mux1/4
  Half Adder7/2(Carry) -> Half Adder/2("B ")
  D Flip-Flop11/1 -> C4/1, Half Adder2/1(A)  "D1"
  D Flip-Flop6/1 -> Half Adder1/1(A)  "D3"
  D Flip-Flop5/1 -> C2/1, Half Adder/1(A)  "D4"
  D Flip-Flop7/1 -> C1/1, Half Adder7/1(A)  "D2"
  NOT/1 -> D Flip-Flop11/3, D Flip-Flop6/3, D Flip-Flop5/3, D Flip-Flop7/3
  D Flip-Flop7/2 -> !C1/1
  D Flip-Flop5/2 -> !C2/1
  D Flip-Flop6/2 -> !C3/1
  D Flip-Flop11/2 -> !C4/1

== system UART/Subsystem1/UART_CON ==
  Data bus : Inport
  Store : Inport  Port=2
  CLK : Inport  Port=3
  CLR : Inport  Port=4
  Demux : Demux  Outputs=8
  Subsystem1 : Subsystem
  Subsystem2 : Subsystem
  Subsystem3 : Subsystem
  Subsystem4 : Subsystem
  Subsystem5 : Subsystem
  Subsystem6 : Subsystem
  Subsystem7 : Subsystem
  Subsystem8 : Subsystem
  EN_RX : Outport
  EN_INT : Outport  Port=2
  wires:
  Demux/4 -> Subsystem2/1(Data)
  Demux/2 -> Subsystem1/1(Data)
  Data bus/1 -> Demux/1
  Store/1 -> Subsystem1/2(Store), Subsystem4/2(Store), Subsystem2/2(Store), Subsystem7/2(Store), Subsystem5/2(Store), Subsystem6/2(Store), Subsystem8/2(Store), Subsystem3/2(Store)
  Demux/5 -> Subsystem7/1(Data)
  Demux/7 -> Subsystem8/1(Data)
  Demux/3 -> Subsystem4/1(Data)
  Demux/6 -> Subsystem5/1(Data)
  Demux/1 -> Subsystem3/1(Data)
  Demux/8 -> Subsystem6/1(Data)
  CLK/1 -> Subsystem1/3(Clock), Subsystem4/3(Clock), Subsystem2/3(Clock), Subsystem7/3(Clock), Subsystem5/3(Clock), Subsystem6/3(Clock), Subsystem8/3(Clock), Subsystem3/3(Clock)
  CLR/1 -> Subsystem8/4(Clear), Subsystem5/4(Clear), Subsystem7/4(Clear), Subsystem2/4(Clear), Subsystem4/4(Clear), Subsystem1/4(Clear), Subsystem3/4(Clear), Subsystem6/4(Clear)
  Subsystem3/1(Q) -> EN_RX/1
  Subsystem1/1(Q) -> EN_INT/1

== system UART/Rx Only/Baudrate Generator/BPS ==
  Data bus : Inport
  Store : Inport  Port=2
  CLK : Inport  Port=3
  CLR : Inport  Port=4
  Demux : Demux  Outputs=8
  Mux : Mux  Inputs=8
  Subsystem1 : Subsystem
  Subsystem2 : Subsystem
  Subsystem3 : Subsystem
  Subsystem4 : Subsystem
  Subsystem5 : Subsystem
  Subsystem6 : Subsystem
  Subsystem7 : Subsystem
  Subsystem8 : Subsystem
  "Q Bus " : Outport
  wires:
  Demux/4 -> Subsystem2/1(Data)
  Mux/1 -> "Q Bus "/1
  Demux/2 -> Subsystem1/1(Data)
  Data bus/1 -> Demux/1
  Subsystem6/1(Q) -> Mux/8
  Store/1 -> Subsystem1/2(Store), Subsystem4/2(Store), Subsystem2/2(Store), Subsystem7/2(Store), Subsystem5/2(Store), Subsystem6/2(Store), Subsystem8/2(Store), Subsystem3/2(Store)
  Demux/5 -> Subsystem7/1(Data)
  Demux/7 -> Subsystem8/1(Data)
  Demux/3 -> Subsystem4/1(Data)
  Subsystem7/1(Q) -> Mux/5
  Demux/6 -> Subsystem5/1(Data)
  Subsystem1/1(Q) -> Mux/2
  Demux/1 -> Subsystem3/1(Data)
  Subsystem3/1(Q) -> Mux/1
  Demux/8 -> Subsystem6/1(Data)
  Subsystem8/1(Q) -> Mux/7
  Subsystem2/1(Q) -> Mux/4
  Subsystem4/1(Q) -> Mux/3
  Subsystem5/1(Q) -> Mux/6
  CLK/1 -> Subsystem1/3(Clock), Subsystem4/3(Clock), Subsystem2/3(Clock), Subsystem7/3(Clock), Subsystem5/3(Clock), Subsystem6/3(Clock), Subsystem8/3(Clock), Subsystem3/3(Clock)
  CLR/1 -> Subsystem8/4(Clear), Subsystem5/4(Clear), Subsystem7/4(Clear), Subsystem2/4(Clear), Subsystem4/4(Clear), Subsystem1/4(Clear), Subsystem3/4(Clear), Subsystem6/4(Clear)

== system UART/Rx Only/Baudrate Generator/BR ==
  Data bus : Inport
  Store : Inport  Port=2
  CLK : Inport  Port=3
  CLR : Inport  Port=4
  Demux : Demux  Outputs=8
  Mux : Mux  Inputs=8
  Subsystem1 : Subsystem
  Subsystem2 : Subsystem
  Subsystem3 : Subsystem
  Subsystem4 : Subsystem
  Subsystem5 : Subsystem
  Subsystem6 : Subsystem
  Subsystem7 : Subsystem
  Subsystem8 : Subsystem
  "Q Bus " : Outport
  wires:
  Demux/4 -> Subsystem2/1(Data)
  Mux/1 -> "Q Bus "/1
  Demux/2 -> Subsystem1/1(Data)
  Data bus/1 -> Demux/1
  Subsystem6/1(Q) -> Mux/8
  Store/1 -> Subsystem1/2(Store), Subsystem4/2(Store), Subsystem2/2(Store), Subsystem7/2(Store), Subsystem5/2(Store), Subsystem6/2(Store), Subsystem8/2(Store), Subsystem3/2(Store)
  Demux/5 -> Subsystem7/1(Data)
  Demux/7 -> Subsystem8/1(Data)
  Demux/3 -> Subsystem4/1(Data)
  Subsystem7/1(Q) -> Mux/5
  Demux/6 -> Subsystem5/1(Data)
  Subsystem1/1(Q) -> Mux/2
  Demux/1 -> Subsystem3/1(Data)
  Subsystem3/1(Q) -> Mux/1
  Demux/8 -> Subsystem6/1(Data)
  Subsystem8/1(Q) -> Mux/7
  Subsystem2/1(Q) -> Mux/4
  Subsystem4/1(Q) -> Mux/3
  Subsystem5/1(Q) -> Mux/6
  CLK/1 -> Subsystem1/3(Clock), Subsystem4/3(Clock), Subsystem2/3(Clock), Subsystem7/3(Clock), Subsystem5/3(Clock), Subsystem6/3(Clock), Subsystem8/3(Clock), Subsystem3/3(Clock)
  CLR/1 -> Subsystem8/4(Clear), Subsystem5/4(Clear), Subsystem7/4(Clear), Subsystem2/4(Clear), Subsystem4/4(Clear), Subsystem1/4(Clear), Subsystem3/4(Clear), Subsystem6/4(Clear)

== system UART/Rx Only/Baudrate Generator/BaudTimer ==
  StoreBR : Inport
  BR_Reg : Inport  Port=2
  Enable : Inport  Port=3
  "CLR " : Inport  Port=4
  StorePS : Inport  Port=5
  TReg : Inport  Port=6
  CLK : Inport  Port=7
  Counter : Subsystem
      settings: PortSchema="{\"entries\":[{\"content\":{\"sides\":[{\"content\":{\"connectorIds\":[\"Out1\",\"In1\",\"In2\"]},\"type\":\"ConnectorPlacement.EquallySpacedRectSide\",\"uuid\":\"d2ca064e-8e65-4383-9509-923487f0994b\"},{\"content\":{\"side\":\"RIGHT\"},\"type\":\"ConnectorPlacement.EquallySpacedRectSide\",\"uuid\":\"c8a688a5-ee2c-4fad-a889-c5e09b1c269e\"},{\"content\":{\"side\":\"TOP\"},\"type\":\"ConnectorPlacement.EquallySpacedRectSide\",\"uuid\":\"2f0d42e7-9a85-4a58-8ec6-3b7b9eab62de\"},{\"content\":{\"side\":\"BOTTOM\"},\"type\":\"ConnectorPlacement.EquallySpacedRectSide\",\"uuid\":\"38510fd4-2d07-404d-8bb1-895f71011c48\"}]},\"type\":\"ConnectorPlacement.EquallySpacedConnector\",\"uuid\":\"c9cdc40f-5296-4098-a99e-74109d120565\"}],\"packageUris\":[\"http://schema.mathworks.com/mf0/Connector/R2020b\"],\"version\":\"1.0\"}"
  Counter1 : Subsystem
      settings: PortSchema="{\"entries\":[{\"content\":{\"sides\":[{\"content\":{\"connectorIds\":[\"Out1\",\"In1\",\"In2\"]},\"type\":\"ConnectorPlacement.EquallySpacedRectSide\",\"uuid\":\"d2ca064e-8e65-4383-9509-923487f0994b\"},{\"content\":{\"side\":\"RIGHT\"},\"type\":\"ConnectorPlacement.EquallySpacedRectSide\",\"uuid\":\"c8a688a5-ee2c-4fad-a889-c5e09b1c269e\"},{\"content\":{\"side\":\"TOP\"},\"type\":\"ConnectorPlacement.EquallySpacedRectSide\",\"uuid\":\"2f0d42e7-9a85-4a58-8ec6-3b7b9eab62de\"},{\"content\":{\"side\":\"BOTTOM\"},\"type\":\"ConnectorPlacement.EquallySpacedRectSide\",\"uuid\":\"38510fd4-2d07-404d-8bb1-895f71011c48\"}]},\"type\":\"ConnectorPlacement.EquallySpacedConnector\",\"uuid\":\"c9cdc40f-5296-4098-a99e-74109d120565\"}],\"packageUris\":[\"http://schema.mathworks.com/mf0/Connector/R2020b\"],\"version\":\"1.0\"}"
  NOT : Logic  Operator=NOT  IconShape=distinctive  AllPortsSameDT=off  OutDataTypeStr=boolean
  OR : Logic  Operator=OR  IconShape=distinctive  AllPortsSameDT=off  OutDataTypeStr=boolean
  OR1 : Logic  Operator=OR  IconShape=distinctive  AllPortsSameDT=off  OutDataTypeStr=boolean
  Prescaler_Controller2 : Subsystem
      settings: PortSchema="{\"entries\":[{\"content\":{\"sides\":[{\"content\":{\"connectorIds\":[\"In1\",\"In2\",\"In3\",\"In4\",\"In5\"]},\"type\":\"ConnectorPlacement.EquallySpacedRectSide\",\"uuid\":\"6170e57a-f155-4328-bd43-dda78d71cb36\"},{\"content\":{\"connectorIds\":[\"Out1\",\"In6\",\"Out2\",\"Out3\"],\"side\":\"RIGHT\"},\"type\":\"ConnectorPlacement.EquallySpacedRectSide\",\"uuid\":\"7c0f968d-cb84-43a5-9c9f-f9604511aa56\"},{\"content\":{\"side\":\"TOP\"},\"type\":\"ConnectorPlacement.EquallySpacedRectSide\",\"uuid\":\"1355edcf-182b-4fd1-b160-c0d036cb64ee\"}]},\"type\":\"ConnectorPlacement.EquallySpacedConnector\",\"uuid\":\"78984415-bd5b-43a2-9907-2f223cffd06f\"}],\"packageUris\":[\"http://schema.mathworks.com/mf0/Connector/R2020b\"],\"version\":\"1.0\"}"
  TController : Subsystem
      settings: PortSchema="{\"entries\":[{\"content\":{\"sides\":[{\"content\":{\"connectorIds\":[\"In1\",\"In2\",\"In3\",\"In4\",\"In5\"]},\"type\":\"ConnectorPlacement.EquallySpacedRectSide\",\"uuid\":\"c3d628b6-8e4a-468e-9cb9-7c1ae20fcc5b\"},{\"content\":{\"connectorIds\":[\"In6\",\"Out1\",\"Out2\",\"Out3\",\"Out4\"],\"side\":\"RIGHT\"},\"type\":\"ConnectorPlacement.EquallySpacedRectSide\",\"uuid\":\"dcacb871-8b22-4c4a-9d8b-9ea734bd0bce\"},{\"content\":{\"side\":\"TOP\"},\"type\":\"ConnectorPlacement.EquallySpacedRectSide\",\"uuid\":\"c4096842-dad0-49fa-9d55-60018b71b534\"}]},\"type\":\"ConnectorPlacement.EquallySpacedConnector\",\"uuid\":\"477c4d17-ed59-4190-8e6d-61e0bddcf33b\"}],\"packageUris\":[\"http://schema.mathworks.com/mf0/Connector/R2020b\"],\"version\":\"1.0\"}"
  B_CLK : Outport
  !B_CLK : Outport  Port=2
  wires:
  Counter/1(TC) -> TController/6(TC)
  TController/4(!B_CLK) -> !B_CLK/1
  Prescaler_Controller2/1(CLK_Next) -> TController/5(CLK)
  NOT/1 -> OR1/2, OR/2
  TController/3(B_CLK) -> B_CLK/1
  Prescaler_Controller2/2(INC) -> Counter1/1(INC)
  StorePS/1 -> Prescaler_Controller2/4(StoreTCON)
  Enable/1 -> TController/4(Enable), Prescaler_Controller2/3(Enable), NOT/1
  OR1/1 -> Counter/2(TC_RST)
  Prescaler_Controller2/3(TC_RST) -> OR/1
  OR/1 -> Counter1/2(TC_RST)
  TController/2(TC_RST) -> OR1/1
  TController/1(INC) -> Counter/1(INC)
  Counter1/1(TC) -> Prescaler_Controller2/6(TC)
  "CLR "/1 -> Prescaler_Controller2/1("CLR "), TController/3("CLR ")
  CLK/1 -> Prescaler_Controller2/5(CLK)
  StoreBR/1 -> TController/1(StoreBR)
  BR_Reg/1 -> TController/2(BR_Reg)
  TReg/1 -> Prescaler_Controller2/2(TReg)

== system UART/Rx Only/Baudrate Generator/BaudTimer1 ==
  StoreBR : Inport
  BR_Reg : Inport  Port=2
  Enable : Inport  Port=3
  "CLR " : Inport  Port=4
  StorePS : Inport  Port=5
  TReg : Inport  Port=6
  CLK : Inport  Port=7
  Counter : Subsystem
      settings: PortSchema="{\"entries\":[{\"content\":{\"sides\":[{\"content\":{\"connectorIds\":[\"Out1\",\"In1\",\"In2\"]},\"type\":\"ConnectorPlacement.EquallySpacedRectSide\",\"uuid\":\"d2ca064e-8e65-4383-9509-923487f0994b\"},{\"content\":{\"side\":\"RIGHT\"},\"type\":\"ConnectorPlacement.EquallySpacedRectSide\",\"uuid\":\"c8a688a5-ee2c-4fad-a889-c5e09b1c269e\"},{\"content\":{\"side\":\"TOP\"},\"type\":\"ConnectorPlacement.EquallySpacedRectSide\",\"uuid\":\"2f0d42e7-9a85-4a58-8ec6-3b7b9eab62de\"},{\"content\":{\"side\":\"BOTTOM\"},\"type\":\"ConnectorPlacement.EquallySpacedRectSide\",\"uuid\":\"38510fd4-2d07-404d-8bb1-895f71011c48\"}]},\"type\":\"ConnectorPlacement.EquallySpacedConnector\",\"uuid\":\"c9cdc40f-5296-4098-a99e-74109d120565\"}],\"packageUris\":[\"http://schema.mathworks.com/mf0/Connector/R2020b\"],\"version\":\"1.0\"}"
  Counter1 : Subsystem
      settings: PortSchema="{\"entries\":[{\"content\":{\"sides\":[{\"content\":{\"connectorIds\":[\"Out1\",\"In1\",\"In2\"]},\"type\":\"ConnectorPlacement.EquallySpacedRectSide\",\"uuid\":\"d2ca064e-8e65-4383-9509-923487f0994b\"},{\"content\":{\"side\":\"RIGHT\"},\"type\":\"ConnectorPlacement.EquallySpacedRectSide\",\"uuid\":\"c8a688a5-ee2c-4fad-a889-c5e09b1c269e\"},{\"content\":{\"side\":\"TOP\"},\"type\":\"ConnectorPlacement.EquallySpacedRectSide\",\"uuid\":\"2f0d42e7-9a85-4a58-8ec6-3b7b9eab62de\"},{\"content\":{\"side\":\"BOTTOM\"},\"type\":\"ConnectorPlacement.EquallySpacedRectSide\",\"uuid\":\"38510fd4-2d07-404d-8bb1-895f71011c48\"}]},\"type\":\"ConnectorPlacement.EquallySpacedConnector\",\"uuid\":\"c9cdc40f-5296-4098-a99e-74109d120565\"}],\"packageUris\":[\"http://schema.mathworks.com/mf0/Connector/R2020b\"],\"version\":\"1.0\"}"
  NOT : Logic  Operator=NOT  IconShape=distinctive  AllPortsSameDT=off  OutDataTypeStr=boolean
  OR : Logic  Operator=OR  IconShape=distinctive  AllPortsSameDT=off  OutDataTypeStr=boolean
  OR1 : Logic  Operator=OR  IconShape=distinctive  AllPortsSameDT=off  OutDataTypeStr=boolean
  Prescaler_Controller1 : Subsystem
      settings: PortSchema="{\"entries\":[{\"content\":{\"sides\":[{\"content\":{\"connectorIds\":[\"In1\",\"In2\",\"In3\",\"In4\",\"In5\"]},\"type\":\"ConnectorPlacement.EquallySpacedRectSide\",\"uuid\":\"82b85bc6-964b-49ee-8a4b-3356bfec1aee\"},{\"content\":{\"connectorIds\":[\"Out1\",\"In6\",\"Out2\",\"Out3\"],\"side\":\"RIGHT\"},\"type\":\"ConnectorPlacement.EquallySpacedRectSide\",\"uuid\":\"8c4af632-7d6e-4ec6-a03e-f6796e56340c\"},{\"content\":{\"side\":\"TOP\"},\"type\":\"ConnectorPlacement.EquallySpacedRectSide\",\"uuid\":\"c668d65a-8355-4e30-8ca9-8213ac4eb35c\"},{\"content\":{\"side\":\"BOTTOM\"},\"type\":\"ConnectorPlacement.EquallySpacedRectSide\",\"uuid\":\"7e82bb91-fecf-4aec-a971-3b22643d51d5\"}]},\"type\":\"ConnectorPlacement.EquallySpacedConnector\",\"uuid\":\"0a0bd963-09d6-4454-bda2-144190581a2a\"}],\"packageUris\":[\"http://schema.mathworks.com/mf0/Connector/R2020b\"],\"version\":\"1.0\"}"
  TController : Subsystem
      settings: PortSchema="{\"entries\":[{\"content\":{\"sides\":[{\"content\":{\"connectorIds\":[\"In1\",\"In2\",\"In3\",\"In4\",\"In5\"]},\"type\":\"ConnectorPlacement.EquallySpacedRectSide\",\"uuid\":\"c3d628b6-8e4a-468e-9cb9-7c1ae20fcc5b\"},{\"content\":{\"connectorIds\":[\"In6\",\"Out1\",\"Out2\",\"Out3\",\"Out4\"],\"side\":\"RIGHT\"},\"type\":\"ConnectorPlacement.EquallySpacedRectSide\",\"uuid\":\"dcacb871-8b22-4c4a-9d8b-9ea734bd0bce\"},{\"content\":{\"side\":\"TOP\"},\"type\":\"ConnectorPlacement.EquallySpacedRectSide\",\"uuid\":\"c4096842-dad0-49fa-9d55-60018b71b534\"}]},\"type\":\"ConnectorPlacement.EquallySpacedConnector\",\"uuid\":\"477c4d17-ed59-4190-8e6d-61e0bddcf33b\"}],\"packageUris\":[\"http://schema.mathworks.com/mf0/Connector/R2020b\"],\"version\":\"1.0\"}"
  B_CLK : Outport
  !B_CLK : Outport  Port=2
  wires:
  Counter/1(TC) -> TController/6(TC)
  TController/4(!B_CLK) -> !B_CLK/1
  Prescaler_Controller1/1(CLK_Next) -> TController/5(CLK)
  NOT/1 -> OR1/2, OR/2
  TController/3(B_CLK) -> B_CLK/1
  Prescaler_Controller1/2(INC) -> Counter1/1(INC)
  StorePS/1 -> Prescaler_Controller1/4(StoreTReg)
  Enable/1 -> TController/4(Enable), NOT/1, Prescaler_Controller1/3(Enable)
  OR1/1 -> Counter/2(TC_RST)
  Prescaler_Controller1/3(TC_RST) -> OR/1
  OR/1 -> Counter1/2(TC_RST)
  TController/2(TC_RST) -> OR1/1
  TController/1(INC) -> Counter/1(INC)
  Counter1/1(TC) -> Prescaler_Controller1/6(TC)
  "CLR "/1 -> TController/3("CLR "), Prescaler_Controller1/1("CLR ")
  CLK/1 -> Prescaler_Controller1/5(CLK)
  StoreBR/1 -> TController/1(StoreBR)
  BR_Reg/1 -> TController/2(BR_Reg)
  TReg/1 -> Prescaler_Controller1/2(TReg)

== system UART/Rx Only/Subsystem1/RX Counter ==
  BC_Reset : Inport
  INC : Inport  Port=2
  Constant : Constant
  D Flip-Flop{5..7,11} (4 alike) : simulink_extras/Flip Flops/D Flip-Flop
  Delay One Step : Delay  DelayLength=1
  Demux : Demux
  Half Adder : Subsystem
      settings: PortSchema="{\"entries\":[{\"content\":{\"sides\":[{\"content\":{\"connectorIds\":[\"In1\"]},\"type\":\"ConnectorPlacement.EquallySpacedRectSide\",\"uuid\":\"d3a7e232-15f2-47a9-a065-9480c81dc57e\"},{\"content\":{\"connectorIds\":[\"Out1\"],\"side\":\"RIGHT\"},\"type\":\"ConnectorPlacement.EquallySpacedRectSide\",\"uuid\":\"e118f150-fee7-4aeb-941e-53c3f02c6791\"},{\"content\":{\"connectorIds\":[\"Out2\"],\"side\":\"TOP\"},\"type\":\"ConnectorPlacement.EquallySpacedRectSide\",\"uuid\":\"6d9038ab-faad-455b-a9c5-8fe0bbf34e51\"},{\"content\":{\"connectorIds\":[\"In2\"],\"side\":\"BOTTOM\"},\"type\":\"ConnectorPlacement.EquallySpacedRectSide\",\"uuid\":\"d09c8d4f-08f3-4c52-88a6-8c6db517fc7a\"}]},\"type\":\"ConnectorPlacement.EquallySpacedConnector\",\"uuid\":\"5bc947ce-f1cd-4957-9186-40c14c78de7d\"}],\"packageUris\":[\"http://schema.mathworks.com/mf0/Connector/R2020b\"],\"version\":\"1.0\"}"
  Half Adder1 : Subsystem
      settings: PortSchema="{\"entries\":[{\"content\":{\"sides\":[{\"content\":{\"connectorIds\":[\"In1\"]},\"type\":\"ConnectorPlacement.EquallySpacedRectSide\",\"uuid\":\"d3a7e232-15f2-47a9-a065-9480c81dc57e\"},{\"content\":{\"connectorIds\":[\"Out1\"],\"side\":\"RIGHT\"},\"type\":\"ConnectorPlacement.EquallySpacedRectSide\",\"uuid\":\"e118f150-fee7-4aeb-941e-53c3f02c6791\"},{\"content\":{\"connectorIds\":[\"Out2\"],\"side\":\"TOP\"},\"type\":\"ConnectorPlacement.EquallySpacedRectSide\",\"uuid\":\"6d9038ab-faad-455b-a9c5-8fe0bbf34e51\"},{\"content\":{\"connectorIds\":[\"In2\"],\"side\":\"BOTTOM\"},\"type\":\"ConnectorPlacement.EquallySpacedRectSide\",\"uuid\":\"d09c8d4f-08f3-4c52-88a6-8c6db517fc7a\"}]},\"type\":\"ConnectorPlacement.EquallySpacedConnector\",\"uuid\":\"5bc947ce-f1cd-4957-9186-40c14c78de7d\"}],\"packageUris\":[\"http://schema.mathworks.com/mf0/Connector/R2020b\"],\"version\":\"1.0\"}"
  Half Adder2 : Subsystem
      settings: PortSchema="{\"entries\":[{\"content\":{\"sides\":[{\"content\":{\"connectorIds\":[\"In1\"]},\"type\":\"ConnectorPlacement.EquallySpacedRectSide\",\"uuid\":\"d3a7e232-15f2-47a9-a065-9480c81dc57e\"},{\"content\":{\"connectorIds\":[\"Out1\"],\"side\":\"RIGHT\"},\"type\":\"ConnectorPlacement.EquallySpacedRectSide\",\"uuid\":\"e118f150-fee7-4aeb-941e-53c3f02c6791\"},{\"content\":{\"connectorIds\":[\"Out2\"],\"side\":\"TOP\"},\"type\":\"ConnectorPlacement.EquallySpacedRectSide\",\"uuid\":\"6d9038ab-faad-455b-a9c5-8fe0bbf34e51\"},{\"content\":{\"connectorIds\":[\"In2\"],\"side\":\"BOTTOM\"},\"type\":\"ConnectorPlacement.EquallySpacedRectSide\",\"uuid\":\"d09c8d4f-08f3-4c52-88a6-8c6db517fc7a\"}]},\"type\":\"ConnectorPlacement.EquallySpacedConnector\",\"uuid\":\"5bc947ce-f1cd-4957-9186-40c14c78de7d\"}],\"packageUris\":[\"http://schema.mathworks.com/mf0/Connector/R2020b\"],\"version\":\"1.0\"}"
  Half Adder7 : Subsystem
      settings: PortSchema="{\"entries\":[{\"content\":{\"sides\":[{\"content\":{\"connectorIds\":[\"In1\"]},\"type\":\"ConnectorPlacement.EquallySpacedRectSide\",\"uuid\":\"d3a7e232-15f2-47a9-a065-9480c81dc57e\"},{\"content\":{\"connectorIds\":[\"Out1\"],\"side\":\"RIGHT\"},\"type\":\"ConnectorPlacement.EquallySpacedRectSide\",\"uuid\":\"e118f150-fee7-4aeb-941e-53c3f02c6791\"},{\"content\":{\"connectorIds\":[\"Out2\"],\"side\":\"TOP\"},\"type\":\"ConnectorPlacement.EquallySpacedRectSide\",\"uuid\":\"6d9038ab-faad-455b-a9c5-8fe0bbf34e51\"},{\"content\":{\"connectorIds\":[\"In2\"],\"side\":\"BOTTOM\"},\"type\":\"ConnectorPlacement.EquallySpacedRectSide\",\"uuid\":\"d09c8d4f-08f3-4c52-88a6-8c6db517fc7a\"}]},\"type\":\"ConnectorPlacement.EquallySpacedConnector\",\"uuid\":\"5bc947ce-f1cd-4957-9186-40c14c78de7d\"}],\"packageUris\":[\"http://schema.mathworks.com/mf0/Connector/R2020b\"],\"version\":\"1.0\"}"
  Mux1 : Mux
  NOT : Logic  Operator=NOT  IconShape=distinctive  AllPortsSameDT=off  OutDataTypeStr=boolean
  C4 : Outport
  !C3 : Outport  Port=2
  !C2 : Outport  Port=3
  C1 : Outport  Port=4
  wires:
  Mux1/1 -> Delay One Step/1
  BC_Reset/1 -> NOT/1
  Delay One Step/1 -> Demux/1
  Demux/4 -> D Flip-Flop7/1
  Demux/3 -> D Flip-Flop5/1
  Demux/2 -> D Flip-Flop6/1
  Demux/1 -> D Flip-Flop11/1
  INC/1 -> D Flip-Flop11/2, D Flip-Flop6/2, D Flip-Flop5/2, D Flip-Flop7/2
  Constant/1 -> Half Adder7/2("B ")
  Half Adder/2(Carry) -> Half Adder1/2("B ")
  Half Adder1/1(Sum) -> Mux1/2
  Half Adder/1(Sum) -> Mux1/3
  Half Adder2/1(Sum) -> Mux1/1
  Half Adder1/2(Carry) -> Half Adder2/2("B ")
  Half Adder7/1(Sum) -> Mux1/4
  Half Adder7/2(Carry) -> Half Adder/2("B ")
  D Flip-Flop11/1 -> C4/1, Half Adder2/1(A)  "D1"
  D Flip-Flop6/1 -> Half Adder1/1(A)  "D3"
  D Flip-Flop5/1 -> Half Adder/1(A)  "D4"
  D Flip-Flop7/1 -> C1/1, Half Adder7/1(A)  "D2"
  NOT/1 -> D Flip-Flop11/3, D Flip-Flop6/3, D Flip-Flop5/3, D Flip-Flop7/3
  D Flip-Flop5/2 -> !C2/1
  D Flip-Flop6/2 -> !C3/1
  D Flip-Flop7/2 -> ?

== system UART/Rx Only/Subsystem1/SIPO RxBuf ==
  Rx : Inport
  CLK : Inport  Port=2
  Constant : Constant
  D Flip-Flop{,1..7} (8 alike) : simulink_extras/Flip Flops/D Flip-Flop
  Mux : Mux  Inputs=8
  RxBuf : Outport
  wires:
  D Flip-Flop4/1 -> D Flip-Flop5/1, Mux/5
  Constant/1 -> D Flip-Flop6/3, D Flip-Flop7/3, D Flip-Flop5/3, D Flip-Flop4/3, D Flip-Flop3/3, D Flip-Flop2/3, D Flip-Flop1/3, D Flip-Flop/3
  Mux/1 -> RxBuf/1
  CLK/1 -> D Flip-Flop1/2, D Flip-Flop2/2, D Flip-Flop3/2, D Flip-Flop4/2, D Flip-Flop5/2, D Flip-Flop6/2, D Flip-Flop7/2, D Flip-Flop/2
  D Flip-Flop6/1 -> D Flip-Flop7/1, Mux/7
  D Flip-Flop1/1 -> D Flip-Flop2/1, Mux/2
  D Flip-Flop2/1 -> D Flip-Flop3/1, Mux/3
  D Flip-Flop3/2 -> ?
  D Flip-Flop3/1 -> D Flip-Flop4/1, Mux/4
  D Flip-Flop7/1 -> Mux/8
  D Flip-Flop/1 -> D Flip-Flop1/1, Mux/1
  D Flip-Flop5/1 -> D Flip-Flop6/1, Mux/6
  D Flip-Flop2/2 -> ?
  Rx/1 -> D Flip-Flop/1
